simulink model "dribbel_v2"  (R2021b)
settings: Solver=FixedStepAuto  StartTime=0.0  StopTime=6  FixedStep=1e-4  MaxStep=1e-3  RelTol=1e-6
InitFcn:
  | dribbel_init_params;
values from neighbouring files (symbols this model uses):
  bd = [modifyPolynomial(polyder(b(1,:)),k); modifyPolynomial(polyder(b(2,:)),k)]    [trajectoryCostFun.m]
  D = m1*(Jvc1'*Jvc1)+m2*(Jvc2'*Jvc2)+m3*(Jvc3'*Jvc3)    [mass_matrix_planar_walker.m]
  g = 9.81    [create_robot_dribbel.m]
undefined symbols (not defined in the file or in its folder): bdd, c2, gamma, k, m, mH, q0, qd0, qdd0, xb
libraries: simulink x10
settings Model: Creator=moham  LastModifiedBy=moham
settings SolverCC: ShapePreserveControl=EnableAll  ZeroCrossAlgorithm=Adaptive

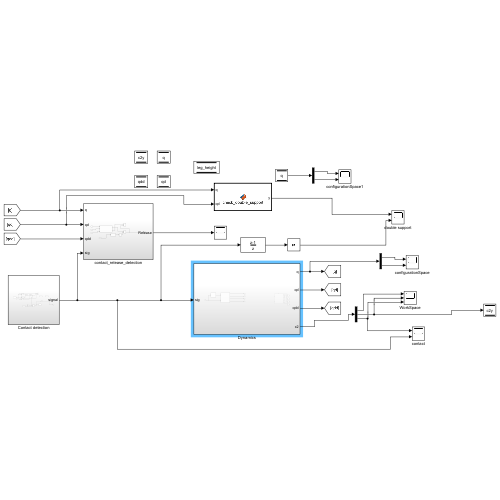
[thumbnail: Simulink's stored preview of the top-level diagram]
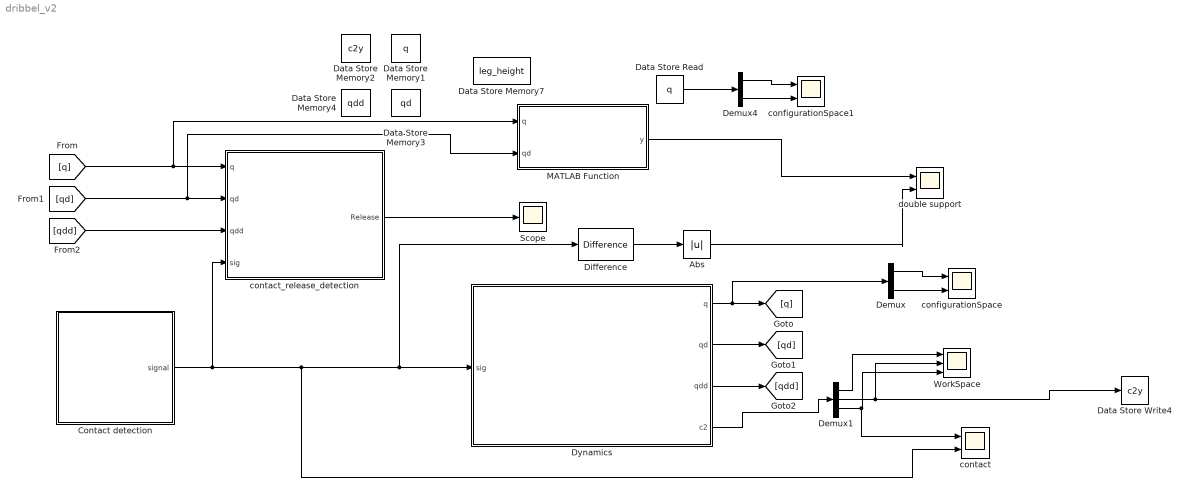
== system dribbel_v2 ==
  Abs : Abs
  Contact detection : Subsystem
  Data Store Memory1 : DataStoreMemory  DataStoreName=q  ReadBeforeWriteMsg=warning  WriteAfterWriteMsg=warning  WriteAfterReadMsg=warning  InitialValue=q0  ShowAdditionalParam=off
  Data Store Memory2 : DataStoreMemory  DataStoreName=c2y  ReadBeforeWriteMsg=warning  WriteAfterWriteMsg=warning  WriteAfterReadMsg=warning  InitialValue=c2(1,1)  ShowAdditionalParam=off
  Data Store Memory3 : DataStoreMemory  DataStoreName=qd  ReadBeforeWriteMsg=warning  WriteAfterWriteMsg=warning  WriteAfterReadMsg=warning  InitialValue=qd0  ShowAdditionalParam=off
  Data Store Memory4 : DataStoreMemory  DataStoreName=qdd  ReadBeforeWriteMsg=warning  WriteAfterWriteMsg=warning  WriteAfterReadMsg=warning  InitialValue=qd0  ShowAdditionalParam=off
  Data Store Memory7 : DataStoreMemory  DataStoreName=leg_height  ReadBeforeWriteMsg=warning  WriteAfterWriteMsg=warning  WriteAfterReadMsg=warning  ShowAdditionalParam=off
  Data Store Read : DataStoreRead  DataStoreName=q  IndexOptions=Index vector (dialog)  Indices=1  OutputSizes=1
  Data Store Write4 : DataStoreWrite  DataStoreName=c2y  IndexOptions=Index vector (dialog)  Indices=1  OutputSizes=1
  Demux : Demux  Outputs=2
  Demux1 : Demux  Outputs=3
  Demux4 : Demux  Outputs=2
  Difference : simulink/Discrete/Difference  ICPrevInput=0.0  OutMin=[]  OutMax=[]  OutDataType=fixdt(1, 16)  OutScaling=2^-10  DoSatur=off
  Dynamics : Subsystem
  MATLAB Function : MATLAB Function  TreatAsAtomicUnit=on
  Scope : Scope
  WorkSpace : Scope  NumInputPorts=3
  configurationSpace : Scope  NumInputPorts=2
  configurationSpace1 : Scope  NumInputPorts=2
  contact : Scope  NumInputPorts=2
  contact_release_detection : Subsystem
  double support : Scope  NumInputPorts=2
  wires:
  Demux1/1 -> WorkSpace/1
  Demux/2 -> configurationSpace/2
  Demux/1 -> configurationSpace/1
  Demux1/3 -> contact/1, WorkSpace/3
  Contact detection/1(signal) -> contact_release_detection/4(sig), contact/2, Difference/1, Dynamics/1(sig)
  Demux4/1 -> configurationSpace1/1
  Demux4/2 -> configurationSpace1/2
  Dynamics/1(q) -> Demux/1, [q]
  Dynamics/4(c2) -> Demux1/1
  Data Store Read/1 -> Demux4/1
  Demux1/2 -> WorkSpace/2, Data Store Write4/1
  Dynamics/2(qd) -> [qd]
  Dynamics/3(qdd) -> [qdd]
  [q] -> MATLAB Function/1(q), contact_release_detection/1(q)
  [qd] -> MATLAB Function/2(qd), contact_release_detection/2(qd)
  [qdd] -> contact_release_detection/3(qdd)
  contact_release_detection/1(Release) -> Scope/1
  MATLAB Function/1(y) -> double support/1
  Difference/1 -> Abs/1
  Abs/1 -> double support/2

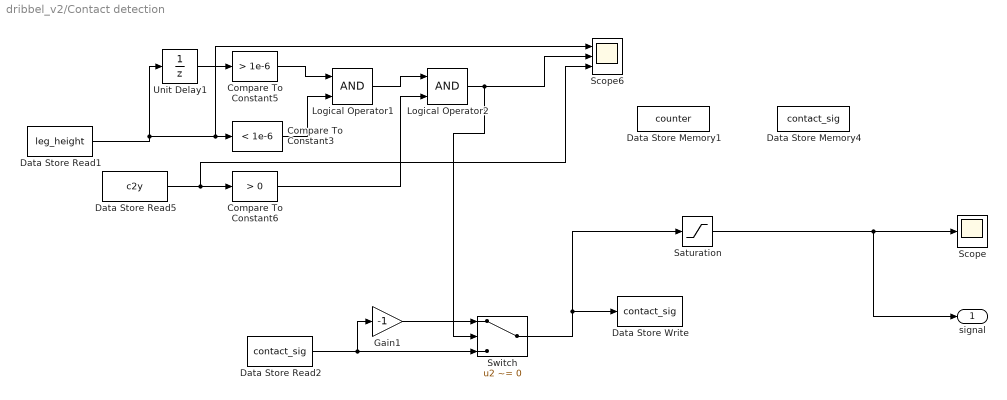
== system dribbel_v2/Contact detection ==
  Compare To Constant3 : simulink/Logic and Bit Operations/Compare To Constant  relop=<  const=1e-6  OutDataTypeStr=uint8  ZeroCross=off
  Compare To Constant5 : simulink/Logic and Bit Operations/Compare To Constant  relop=>  const=1e-6  OutDataTypeStr=uint8  ZeroCross=off
  Compare To Constant6 : simulink/Logic and Bit Operations/Compare To Constant  relop=>  const=0  OutDataTypeStr=uint8  ZeroCross=off
  Data Store Memory1 : DataStoreMemory  DataStoreName=counter  ReadBeforeWriteMsg=warning  WriteAfterWriteMsg=warning  WriteAfterReadMsg=warning  ShowAdditionalParam=off
  Data Store Memory4 : DataStoreMemory  DataStoreName=contact_sig  ReadBeforeWriteMsg=warning  WriteAfterWriteMsg=warning  WriteAfterReadMsg=warning  InitialValue=1  ShowAdditionalParam=off
  Data Store Read1 : DataStoreRead  DataStoreName=leg_height  IndexOptions=Index vector (dialog)  Indices=1  OutputSizes=1
  Data Store Read2 : DataStoreRead  DataStoreName=contact_sig  IndexOptions=Index vector (dialog)  Indices=1  OutputSizes=1
  Data Store Read5 : DataStoreRead  DataStoreName=c2y  IndexOptions=Index vector (dialog)  Indices=1  OutputSizes=1
  Data Store Write : DataStoreWrite  DataStoreName=contact_sig  IndexOptions=Index vector (dialog)  Indices=1  OutputSizes=1
  Gain1 : Gain  Gain=-1
  Logical Operator1 : Logic  AllPortsSameDT=off  OutDataTypeStr=boolean
  Logical Operator2 : Logic  AllPortsSameDT=off  OutDataTypeStr=boolean
  Saturation : Saturate  UpperLimit=1  LowerLimit=0  ZeroCross=off
  Scope : Scope
  Scope6 : Scope  NumInputPorts=3
  Switch : Switch  Criteria=u2 ~= 0  Threshold=0.5  ZeroCross=off
  Unit Delay1 : UnitDelay  SampleTime=-1  HasFrameUpgradeWarning=on
  signal : Outport
  wires:
  Gain1/1 -> Switch/1
  Data Store Read2/1 -> Gain1/1, Switch/3
  Switch/1 -> Saturation/1, Data Store Write/1
  Unit Delay1/1 -> Compare To Constant5/1
  Compare To Constant5/1 -> Logical Operator1/1
  Compare To Constant3/1 -> Logical Operator1/2
  Data Store Read5/1 -> Scope6/3, Compare To Constant6/1
  Compare To Constant6/1 -> Logical Operator2/2
  Logical Operator1/1 -> Logical Operator2/1
  Logical Operator2/1 -> Switch/2, Scope6/2
  Data Store Read1/1 -> Unit Delay1/1, Scope6/1, Compare To Constant3/1
  Saturation/1 -> signal/1, Scope/1

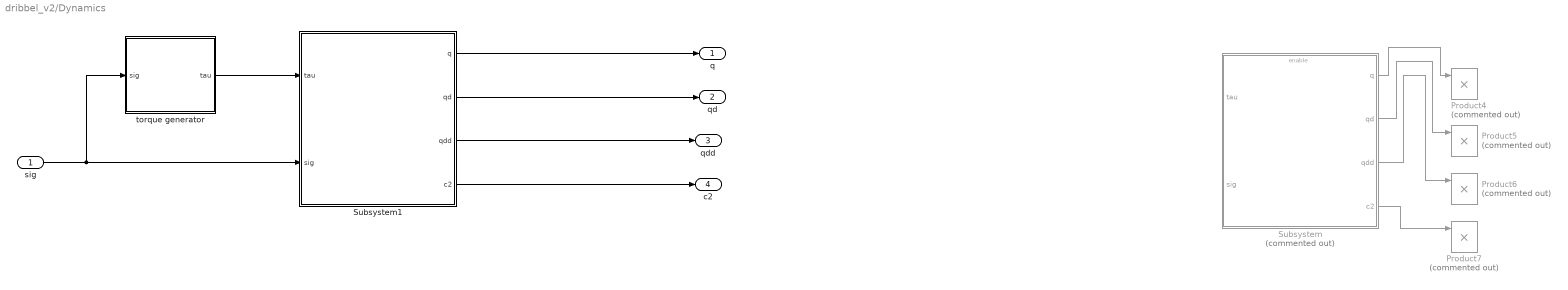
== system dribbel_v2/Dynamics ==
  sig : Inport
  Product{4..7} (4 alike) : Product  Commented=on
  Subsystem : Subsystem  Commented=on
  Subsystem1 : Subsystem
  torque generator : Subsystem
  q : Outport
  qd : Outport  Port=2
  qdd : Outport  Port=3
  c2 : Outport  Port=4
  wires:
  Subsystem1/1(q) -> q/1
  sig/1 -> torque generator/1(sig), Subsystem1/2(sig)
  Subsystem1/4(c2) -> c2/1
  Subsystem/1(q) -> Product4/1
  Subsystem/2(qd) -> Product5/1
  Subsystem/3(qdd) -> Product6/1
  Subsystem/4(c2) -> Product7/1
  Subsystem1/2(qd) -> qd/1
  Subsystem1/3(qdd) -> qdd/1
  torque generator/1(tau) -> Subsystem1/1(tau)

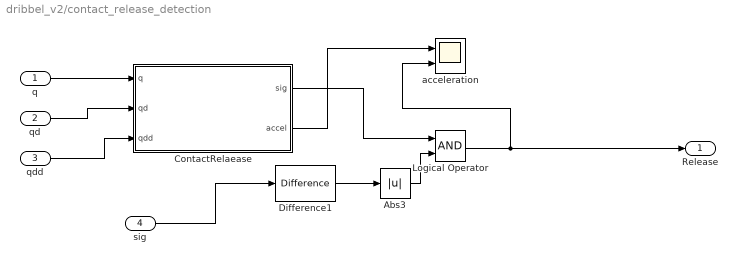
== system dribbel_v2/contact_release_detection ==
  q : Inport
  qd : Inport  Port=2
  qdd : Inport  Port=3
  sig : Inport  Port=4
  Abs3 : Abs
  ContactRelaease : Subsystem
  Difference1 : simulink/Discrete/Difference  ICPrevInput=0.0  OutMin=[]  OutMax=[]  OutDataType=fixdt(1, 16)  OutScaling=2^-10  DoSatur=off
  Logical Operator : Logic  AllPortsSameDT=off  OutDataTypeStr=boolean
  acceleration : Scope  NumInputPorts=2
  Release : Outport
  wires:
  Abs3/1 -> Logical Operator/2
  qd/1 -> ContactRelaease/2(qd)
  ContactRelaease/1(sig) -> Logical Operator/1
  q/1 -> ContactRelaease/1(q)
  Difference1/1 -> Abs3/1
  qdd/1 -> ContactRelaease/3(qdd)
  Logical Operator/1 -> acceleration/2, Release/1
  sig/1 -> Difference1/1
  ContactRelaease/2(accel) -> acceleration/1

== system dribbel_v2/Dynamics/Subsystem ==
  tau : Inport
  sig : Inport  Port=2
  Enable : EnablePort
  Dynamics1 : Subsystem
  Product : Product
  q : Outport
  qd : Outport  Port=2
  qdd : Outport  Port=3
  c2 : Outport  Port=4
  wires:
  Dynamics1/2(qd) -> qd/1
  Dynamics1/4(c2) -> c2/1
  tau/1 -> Dynamics1/2(tau)
  Dynamics1/3(qdd) -> qdd/1
  Dynamics1/1(q) -> Product/2
  Product/1 -> q/1
  sig/1 -> Product/1, Dynamics1/1(sig)

== system dribbel_v2/Dynamics/Subsystem1 ==
  tau : Inport
  sig : Inport  Port=2
  Dynamics : Subsystem
  q : Outport
  qd : Outport  Port=2
  qdd : Outport  Port=3
  c2 : Outport  Port=4
  wires:
  Dynamics/4(c2) -> c2/1
  tau/1 -> Dynamics/2(tau)
  Dynamics/2(qd) -> qd/1
  Dynamics/3(qdd) -> qdd/1
  Dynamics/1(q) -> q/1
  sig/1 -> Dynamics/1(sig)

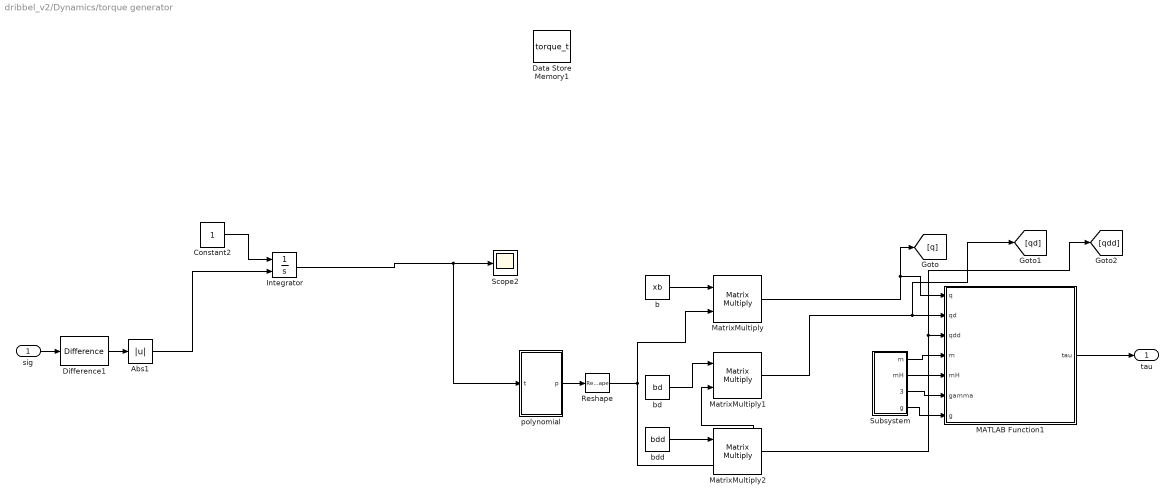
== system dribbel_v2/Dynamics/torque generator ==
  sig : Inport
  Abs1 : Abs
  Constant2 : Constant
  Data Store Memory1 : DataStoreMemory  DataStoreName=torque_t  ReadBeforeWriteMsg=warning  WriteAfterWriteMsg=warning  WriteAfterReadMsg=warning  ShowAdditionalParam=off
  Difference1 : simulink/Discrete/Difference  ICPrevInput=1  OutMin=[]  OutMax=[]  OutDataType=fixdt(1, 16)  OutScaling=2^-10  DoSatur=off
  Integrator : Integrator  ExternalReset=rising
  MATLAB Function1 : MATLAB Function  TreatAsAtomicUnit=on
  MatrixMultiply : Product  Multiplication=Matrix(*)
  MatrixMultiply1 : Product  Multiplication=Matrix(*)
  MatrixMultiply2 : Product  Multiplication=Matrix(*)
  Reshape : Reshape  OutputDimensionality=Column vector (2-D)
  Scope2 : Scope
  Subsystem : Subsystem
  b : Constant  Value=xb
  bd : Constant  Value=bd
  bdd : Constant  Value=bdd
  polynomial : Subsystem
  tau : Outport
  wires:
  bd/1 -> MatrixMultiply1/1
  bdd/1 -> MatrixMultiply2/1
  b/1 -> MatrixMultiply/1
  Subsystem/1(m) -> MATLAB Function1/4(m)
  Subsystem/2(mH) -> MATLAB Function1/5(mH)
  Subsystem/3(gamma) -> MATLAB Function1/6(gamma)
  Subsystem/4(g) -> MATLAB Function1/7(g)
  Reshape/1 -> MatrixMultiply/2, MatrixMultiply1/2, MatrixMultiply2/2
  polynomial/1(p) -> Reshape/1
  sig/1 -> Difference1/1
  Difference1/1 -> Abs1/1
  Abs1/1 -> Integrator/2
  MATLAB Function1/1(tau) -> tau/1
  MatrixMultiply/1 -> [q], MATLAB Function1/1(q)
  MatrixMultiply1/1 -> [qd], MATLAB Function1/2(qd)
  MatrixMultiply2/1 -> [qdd], MATLAB Function1/3(qdd)
  Integrator/1 -> polynomial/1(t), Scope2/1
  Constant2/1 -> Integrator/1

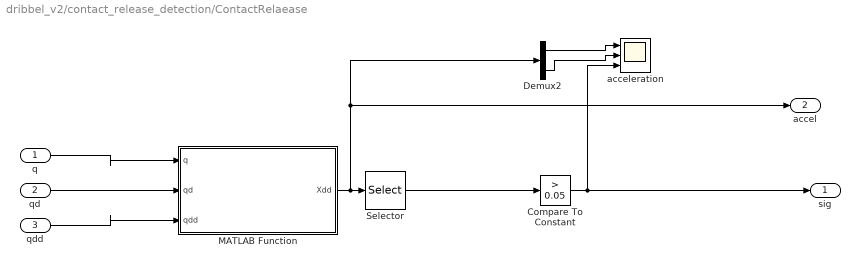
== system dribbel_v2/contact_release_detection/ContactRelaease ==
  q : Inport
  qd : Inport  Port=2
  qdd : Inport  Port=3
  Compare To Constant : simulink/Logic and Bit Operations/Compare To Constant  relop=>  const=0.05  OutDataTypeStr=boolean
  Demux2 : Demux  Outputs=2
  MATLAB Function : MATLAB Function  TreatAsAtomicUnit=on
  Selector : Selector  InputPortWidth=2  IndexOptions=Index vector (dialog)  Indices=2  OutputSizes=1
  acceleration : Scope  NumInputPorts=3
  sig : Outport
  accel : Outport  Port=2
  wires:
  qd/1 -> MATLAB Function/2(qd)
  qdd/1 -> MATLAB Function/3(qdd)
  q/1 -> MATLAB Function/1(q)
  MATLAB Function/1(Xdd) -> accel/1, Demux2/1, Selector/1
  Selector/1 -> Compare To Constant/1
  Demux2/1 -> acceleration/1
  Demux2/2 -> acceleration/2
  Compare To Constant/1 -> sig/1, acceleration/3

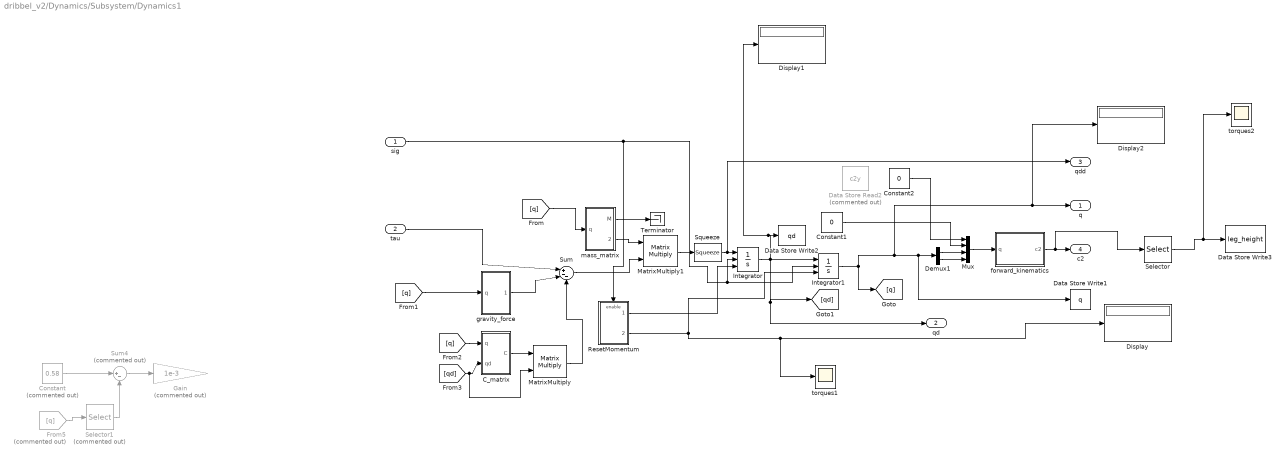
== system dribbel_v2/Dynamics/Subsystem/Dynamics1 ==
  sig : Inport
  tau : Inport  Port=2
  C_matrix : Subsystem
  Constant : Constant  Commented=on  Value=0.58
  Constant1 : Constant  Value=0
  Constant2 : Constant  Value=0
  Data Store Read2 : DataStoreRead  Commented=on  DataStoreName=c2y  IndexOptions=Index vector (dialog)  Indices=1  OutputSizes=1
  Data Store Write1 : DataStoreWrite  DataStoreName=q  IndexOptions=Index vector (dialog)  Indices=1  OutputSizes=1
  Data Store Write2 : DataStoreWrite  DataStoreName=qd  IndexOptions=Index vector (dialog)  Indices=1  OutputSizes=1
  Data Store Write3 : DataStoreWrite  DataStoreName=leg_height  IndexOptions=Index vector (dialog)  Indices=1  OutputSizes=1
  Demux1 : Demux  Outputs=2
  Display : Display
  Display1 : Display
  Display2 : Display
  From5 : From  Commented=on  GotoTag=q
  Gain : Gain  Commented=on  Gain=1e-3
  Integrator : Integrator  ExternalReset=rising  InitialConditionSource=external  InitialCondition=qd0
  Integrator1 : Integrator  ExternalReset=rising  InitialConditionSource=external  InitialCondition=q0
  MatrixMultiply : Product  Multiplication=Matrix(*)
  MatrixMultiply1 : Product  Multiplication=Matrix(*)
  Mux : Mux
  ResetMomentum : Subsystem
  Selector : Selector  InputPortWidth=3  IndexOptions=Index vector (dialog)  Indices=3  OutputSizes=1
  Selector1 : Selector  Commented=on  InputPortWidth=2  IndexOptions=Index vector (dialog)  Indices=2  OutputSizes=1
  Squeeze : Squeeze
  Sum : Sum  Inputs=|+--
  Sum4 : Sum  Commented=on  Inputs=|+-
  Terminator : Terminator
  forward_kinematics : MATLAB Function  TreatAsAtomicUnit=on
  gravity_force : Subsystem
  mass_matrix : Subsystem
  torques1 : Scope
  torques2 : Scope
  q : Outport
  qd : Outport  Port=2
  qdd : Outport  Port=3
  c2 : Outport  Port=4
  wires:
  Constant2/1 -> Mux/1
  C_matrix/1(C) -> MatrixMultiply/1
  mass_matrix/1(M) -> Terminator/1
  mass_matrix/2(M_inv) -> MatrixMultiply1/1
  Sum/1 -> MatrixMultiply1/2
  gravity_force/1(dvdq) -> Sum/2
  MatrixMultiply1/1 -> Squeeze/1
  [qd] -> MatrixMultiply/2, C_matrix/2(qd)
  [q] -> mass_matrix/1(q)
  [q] -> C_matrix/1(q)
  MatrixMultiply/1 -> Sum/3
  [q] -> gravity_force/1(q)
  Squeeze/1 -> Integrator/1, qdd/1
  Demux1/2 -> Mux/4
  Demux1/1 -> Mux/3
  forward_kinematics/1(c2) -> Selector/1, c2/1
  Integrator/1 -> qd/1, [qd], Display1/1, Data Store Write2/1, Integrator1/1
  Mux/1 -> forward_kinematics/1(q)
  Integrator1/1 -> [q], Display2/1, q/1, Demux1/1, Data Store Write1/1
  Selector/1 -> torques2/1, Data Store Write3/1
  Constant1/1 -> Mux/2
  Selector1/1 -> Sum4/2
  From5/1 -> Selector1/1
  Sum4/1 -> Gain/1
  Constant/1 -> Sum4/1
  tau/1 -> Sum/1
  ResetMomentum/2(q_new) -> Integrator1/3, Display/1, torques1/1
  sig/1 -> ResetMomentum/Enable, Integrator1/2, Integrator/2
  ResetMomentum/1(qd_new) -> Integrator/3

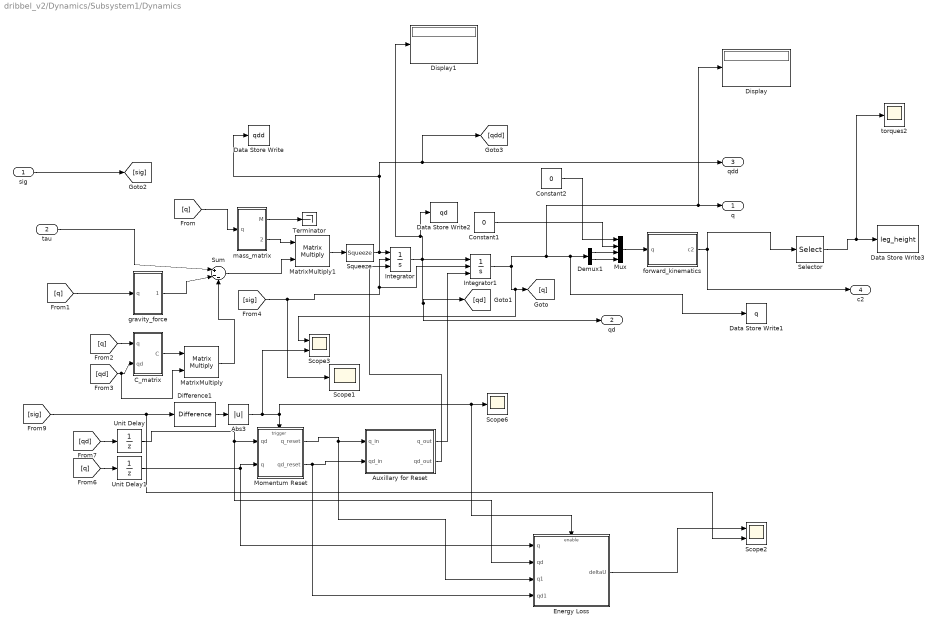
== system dribbel_v2/Dynamics/Subsystem1/Dynamics ==
  sig : Inport
  tau : Inport  Port=2
  Abs3 : Abs
  Auxillary for Reset : Subsystem
  C_matrix : Subsystem
  Constant1 : Constant  Value=0
  Constant2 : Constant  Value=0
  Data Store Write : DataStoreWrite  DataStoreName=qdd  IndexOptions=Index vector (dialog)  Indices=1  OutputSizes=1
  Data Store Write1 : DataStoreWrite  DataStoreName=q  IndexOptions=Index vector (dialog)  Indices=1  OutputSizes=1
  Data Store Write2 : DataStoreWrite  DataStoreName=qd  IndexOptions=Index vector (dialog)  Indices=1  OutputSizes=1
  Data Store Write3 : DataStoreWrite  DataStoreName=leg_height  IndexOptions=Index vector (dialog)  Indices=1  OutputSizes=1
  Demux1 : Demux  Outputs=2
  Difference1 : simulink/Discrete/Difference  ICPrevInput=0.0  OutMin=[]  OutMax=[]  OutDataType=fixdt(1, 16)  OutScaling=2^-10  DoSatur=off
  Display : Display
  Display1 : Display
  Energy Loss : Subsystem  TreatAsAtomicUnit=on
  Integrator : Integrator  ExternalReset=either  InitialConditionSource=external  InitialCondition=qd0  ZeroCross=off
  Integrator1 : Integrator  ExternalReset=either  InitialConditionSource=external  InitialCondition=q0
  MatrixMultiply : Product  Multiplication=Matrix(*)
  MatrixMultiply1 : Product  Multiplication=Matrix(*)
  Momentum Reset : Subsystem
  Mux : Mux
  Scope1 : Scope
  Scope2 : Scope  NumInputPorts=2
  Scope3 : Scope  NumInputPorts=2
  Scope6 : Scope
  Selector : Selector  InputPortWidth=3  IndexOptions=Index vector (dialog)  Indices=3  OutputSizes=1
  Squeeze : Squeeze
  Sum : Sum  Inputs=|+--
  Terminator : Terminator
  Unit Delay : UnitDelay  InitialCondition=qd0  SampleTime=-1  HasFrameUpgradeWarning=on
  Unit Delay1 : UnitDelay  InitialCondition=q0  SampleTime=-1  HasFrameUpgradeWarning=on
  forward_kinematics : MATLAB Function  TreatAsAtomicUnit=on
  gravity_force : Subsystem
  mass_matrix : Subsystem
  torques2 : Scope
  q : Outport
  qd : Outport  Port=2
  qdd : Outport  Port=3
  c2 : Outport  Port=4
  wires:
  tau/1 -> Sum/1
  Constant1/1 -> Mux/2
  Selector/1 -> Data Store Write3/1, torques2/1
  Mux/1 -> forward_kinematics/1(q)
  Integrator/1 -> Integrator1/1, Data Store Write2/1, Display1/1, [qd], qd/1
  forward_kinematics/1(c2) -> c2/1, Selector/1
  Demux1/1 -> Mux/3
  Demux1/2 -> Mux/4
  Squeeze/1 -> Data Store Write/1, [qdd], qdd/1, Integrator/1
  [q] -> gravity_force/1(q)
  MatrixMultiply/1 -> Sum/3
  [q] -> C_matrix/1(q)
  [q] -> mass_matrix/1(q)
  [qd] -> C_matrix/2(qd), MatrixMultiply/2
  MatrixMultiply1/1 -> Squeeze/1
  gravity_force/1(dvdq) -> Sum/2
  Sum/1 -> MatrixMultiply1/2
  mass_matrix/2(M_inv) -> MatrixMultiply1/1
  mass_matrix/1(M) -> Terminator/1
  C_matrix/1(C) -> MatrixMultiply/1
  Constant2/1 -> Mux/1
  Integrator1/1 -> Data Store Write1/1, Demux1/1, q/1, Display/1, Scope3/1, [q]
  sig/1 -> [sig]
  [q] -> Unit Delay1/1
  [sig] -> Scope2/2, Difference1/1
  Difference1/1 -> Abs3/1
  Momentum Reset/1(q_reset) -> Energy Loss/3(q1), Auxillary for Reset/1(q_in)
  Auxillary for Reset/1(q_out) -> Integrator1/3
  Auxillary for Reset/2(qd_out) -> Integrator/3
  [sig] -> Scope1/1, Integrator1/2, Integrator/2
  Unit Delay/1 -> Energy Loss/2(qd), Momentum Reset/1(qd)
  Unit Delay1/1 -> Momentum Reset/2(q), Energy Loss/1(q)
  [qd] -> Unit Delay/1
  Energy Loss/1(deltaU) -> Scope2/1
  Momentum Reset/2(qd_reset) -> Auxillary for Reset/2(qd_in), Energy Loss/4(qd1)
  Abs3/1 -> Scope3/2, Energy Loss/Enable, Scope6/1, Momentum Reset/Trigger

== system dribbel_v2/Dynamics/torque generator/Subsystem ==
  Constan2 : Constant  Value=mH
  Constant : Constant  Value=g
  Constant1 : Constant  Value=gamma
  leg_mass2 : Constant  Value=m
  m : Outport
  mH : Outport  Port=2
  gamma : Outport  Port=3
  g : Outport  Port=4
  wires:
  Constan2/1 -> mH/1
  Constant1/1 -> gamma/1
  Constant/1 -> g/1
  leg_mass2/1 -> m/1

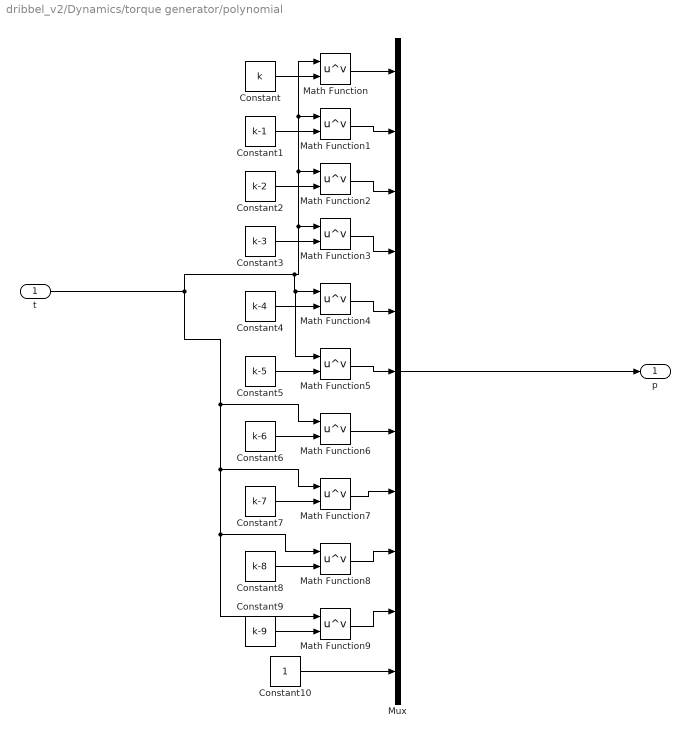
== system dribbel_v2/Dynamics/torque generator/polynomial ==
  t : Inport
  Constant : Constant  Value=k
  Constant1 : Constant  Value=k-1
  Constant10 : Constant
  Constant2 : Constant  Value=k-2
  Constant3 : Constant  Value=k-3
  Constant4 : Constant  Value=k-4
  Constant5 : Constant  Value=k-5
  Constant6 : Constant  Value=k-6
  Constant7 : Constant  Value=k-7
  Constant8 : Constant  Value=k-8
  Constant9 : Constant  Value=k-9
  Math Function{,1..9} (10 alike) : Math  Operator=pow  SaturateOnIntegerOverflow=on
  Mux : Mux  Inputs=11
  p : Outport
  wires:
  Constant/1 -> Math Function/2
  Constant1/1 -> Math Function1/2
  Constant2/1 -> Math Function2/2
  Constant3/1 -> Math Function3/2
  Constant4/1 -> Math Function4/2
  Constant5/1 -> Math Function5/2
  Constant6/1 -> Math Function6/2
  Constant7/1 -> Math Function7/2
  Constant8/1 -> Math Function8/2
  Constant9/1 -> Math Function9/2
  t/1 -> Math Function5/1, Math Function4/1, Math Function3/1, Math Function2/1, Math Function1/1, Math Function/1, Math Function9/1, Math Function8/1, Math Function7/1, Math Function6/1
  Math Function/1 -> Mux/1
  Math Function1/1 -> Mux/2
  Math Function2/1 -> Mux/3
  Math Function3/1 -> Mux/4
  Math Function4/1 -> Mux/5
  Math Function5/1 -> Mux/6
  Math Function6/1 -> Mux/7
  Math Function7/1 -> Mux/8
  Math Function8/1 -> Mux/9
  Math Function9/1 -> Mux/10
  Mux/1 -> p/1
  Constant10/1 -> Mux/11

== system dribbel_v2/Dynamics/Subsystem/Dynamics1/C_matrix ==
  q : Inport
  qd : Inport  Port=2
  C_matrix : MATLAB Function  TreatAsAtomicUnit=on
  leg_mass1 : Constant  Value=m
  C : Outport
  wires:
  leg_mass1/1 -> C_matrix/3(m)
  C_matrix/1(C) -> C/1
  q/1 -> C_matrix/1(q)
  qd/1 -> C_matrix/2(qd)

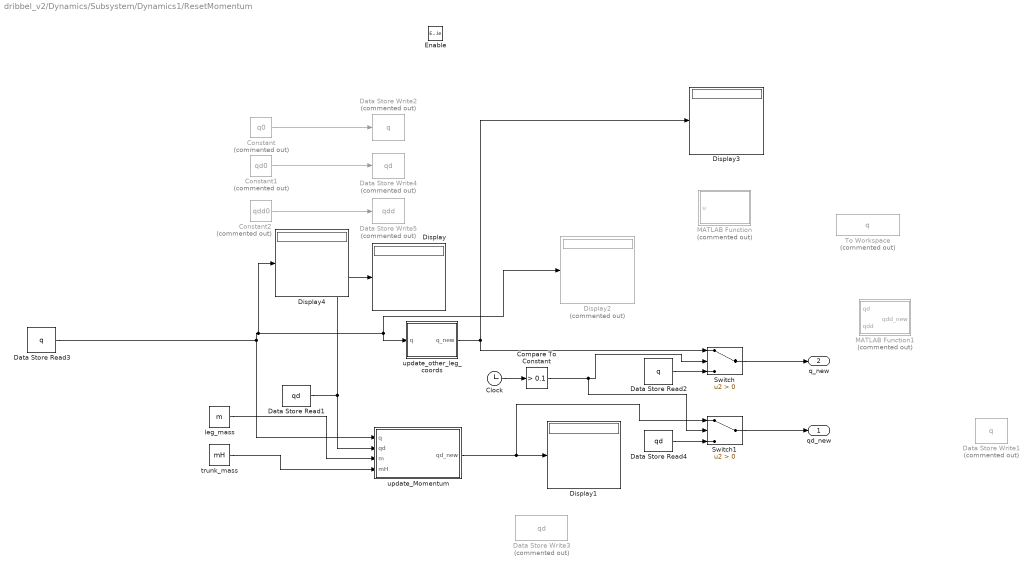
== system dribbel_v2/Dynamics/Subsystem/Dynamics1/ResetMomentum ==
  Enable : EnablePort  StatesWhenEnabling=reset  ZeroCross=off
  Clock : Clock
  Compare To Constant : simulink/Logic and Bit Operations/Compare To Constant  relop=>  const=0.1  OutDataTypeStr=boolean
  Constant : Constant  Commented=on  Value=q0
  Constant1 : Constant  Commented=on  Value=qd0
  Constant2 : Constant  Commented=on  Value=qdd0
  Data Store Read1 : DataStoreRead  DataStoreName=qd  IndexOptions=Index vector (dialog)  Indices=1  OutputSizes=1
  Data Store Read2 : DataStoreRead  DataStoreName=q  IndexOptions=Index vector (dialog)  Indices=1  OutputSizes=1
  Data Store Read3 : DataStoreRead  DataStoreName=q  IndexOptions=Index vector (dialog)  Indices=1  OutputSizes=1
  Data Store Read4 : DataStoreRead  DataStoreName=qd  IndexOptions=Index vector (dialog)  Indices=1  OutputSizes=1
  Data Store Write1 : DataStoreWrite  Commented=on  DataStoreName=q  IndexOptions=Index vector (dialog)  Indices=1  OutputSizes=1
  Data Store Write2 : DataStoreWrite  Commented=on  DataStoreName=q  IndexOptions=Index vector (dialog)  Indices=1  OutputSizes=1
  Data Store Write3 : DataStoreWrite  Commented=on  DataStoreName=qd  IndexOptions=Index vector (dialog)  Indices=1  OutputSizes=1
  Data Store Write4 : DataStoreWrite  Commented=on  DataStoreName=qd  IndexOptions=Index vector (dialog)  Indices=1  OutputSizes=1
  Data Store Write5 : DataStoreWrite  Commented=on  DataStoreName=qdd  IndexOptions=Index vector (dialog)  Indices=1  OutputSizes=1
  Display{,1,3..4} (4 alike) : Display
  Display2 : Display  Commented=on
  MATLAB Function : MATLAB Function  Commented=on  TreatAsAtomicUnit=on
  MATLAB Function1 : MATLAB Function  Commented=on  TreatAsAtomicUnit=on
  Switch : Switch  Criteria=u2 > Threshold
  Switch1 : Switch  Criteria=u2 > Threshold
  To Workspace : ToWorkspace  Commented=on  VariableName=q  SaveFormat=Timeseries  SampleTime=-1
  leg_mass : Constant  Value=m
  trunk_mass : Constant  Value=mH
  update_Momentum : MATLAB Function  TreatAsAtomicUnit=on
  update_other_leg_coords : MATLAB Function  TreatAsAtomicUnit=on
  qd_new : Outport
  q_new : Outport  Port=2
  wires:
  update_Momentum/1(qd_new) -> Switch1/1, Display1/1
  update_other_leg_coords/1(q_new) -> Display3/1, Switch/1
  Constant2/1 -> Data Store Write5/1
  Constant1/1 -> Data Store Write4/1
  Constant/1 -> Data Store Write2/1
  leg_mass/1 -> update_Momentum/3(m)
  Data Store Read1/1 -> update_Momentum/2(qd), Display/1
  trunk_mass/1 -> update_Momentum/4(mH)
  Data Store Read2/1 -> Switch/3
  Switch1/1 -> qd_new/1
  Data Store Read4/1 -> Switch1/3
  Clock/1 -> Compare To Constant/1
  Compare To Constant/1 -> Switch1/2, Switch/2
  Switch/1 -> q_new/1
  Data Store Read3/1 -> Display4/1, update_other_leg_coords/1(q), Display2/1, update_Momentum/1(q)

== system dribbel_v2/Dynamics/Subsystem/Dynamics1/gravity_force ==
  q : Inport
  Constant : Constant  Value=g
  Graitational_Force : MATLAB Function  TreatAsAtomicUnit=on
  gamma : Constant  Value=gamma
  leg_mass2 : Constant  Value=m
  trunk_mass2 : Constant  Value=mH
  dvdq : Outport
  wires:
  trunk_mass2/1 -> Graitational_Force/3(mH)
  leg_mass2/1 -> Graitational_Force/2(m)
  gamma/1 -> Graitational_Force/4(gamma)
  Graitational_Force/1(dvdq) -> dvdq/1
  q/1 -> Graitational_Force/1(q)
  Constant/1 -> Graitational_Force/5(g)

== system dribbel_v2/Dynamics/Subsystem/Dynamics1/mass_matrix ==
  q : Inport
  Mass_Matrix : MATLAB Function  TreatAsAtomicUnit=on
  leg_mass : Constant  Value=m
  trunk_mass : Constant  Value=mH
  M : Outport
  M_inv : Outport  Port=2
  wires:
  Mass_Matrix/2(M_inv) -> M_inv/1
  leg_mass/1 -> Mass_Matrix/2(m)
  q/1 -> Mass_Matrix/1(q)
  Mass_Matrix/1(M) -> M/1
  trunk_mass/1 -> Mass_Matrix/3(mH)

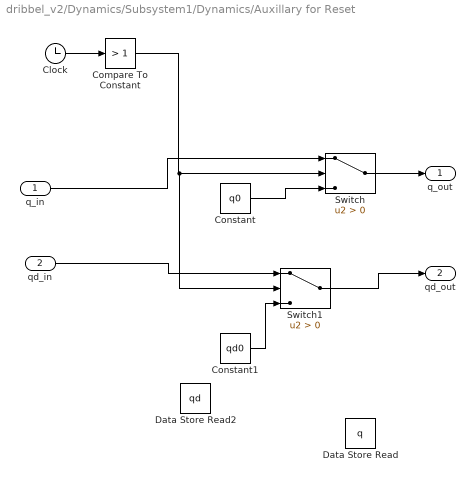
== system dribbel_v2/Dynamics/Subsystem1/Dynamics/Auxillary for Reset ==
  q_in : Inport
  qd_in : Inport  Port=2
  Clock : Clock
  Compare To Constant : simulink/Logic and Bit Operations/Compare To Constant  relop=>  const=1  OutDataTypeStr=boolean
  Constant : Constant  Value=q0
  Constant1 : Constant  Value=qd0
  Data Store Read : DataStoreRead  DataStoreName=q  IndexOptions=Index vector (dialog)  Indices=1  OutputSizes=1
  Data Store Read2 : DataStoreRead  DataStoreName=qd  IndexOptions=Index vector (dialog)  Indices=1  OutputSizes=1
  Switch : Switch  Criteria=u2 > Threshold
  Switch1 : Switch  Criteria=u2 > Threshold
  q_out : Outport
  qd_out : Outport  Port=2
  wires:
  Clock/1 -> Compare To Constant/1
  q_in/1 -> Switch/1
  Compare To Constant/1 -> Switch1/2, Switch/2
  qd_in/1 -> Switch1/1
  Constant/1 -> Switch/3
  Constant1/1 -> Switch1/3
  Switch/1 -> q_out/1
  Switch1/1 -> qd_out/1

== system dribbel_v2/Dynamics/Subsystem1/Dynamics/C_matrix ==
  q : Inport
  qd : Inport  Port=2
  C_matrix : MATLAB Function  TreatAsAtomicUnit=on
  leg_mass1 : Constant  Value=m
  C : Outport
  wires:
  qd/1 -> C_matrix/2(qd)
  q/1 -> C_matrix/1(q)
  C_matrix/1(C) -> C/1
  leg_mass1/1 -> C_matrix/3(m)

== system dribbel_v2/Dynamics/Subsystem1/Dynamics/Energy Loss ==
  q : Inport
  qd : Inport  Port=2
  q1 : Inport  Port=3
  qd1 : Inport  Port=4
  Enable : EnablePort
  Energy After impact : MATLAB Function  TreatAsAtomicUnit=on
  Energy before impact : MATLAB Function  TreatAsAtomicUnit=on
  Sum : Sum  Inputs=-+|
  deltaU : Outport
  wires:
  q/1 -> Energy before impact/1(q)
  qd/1 -> Energy before impact/2(qd)
  Energy before impact/1(K) -> Sum/1
  qd1/1 -> Energy After impact/2(qd)
  q1/1 -> Energy After impact/1(q)
  Energy After impact/1(K) -> Sum/2
  Sum/1 -> deltaU/1

== system dribbel_v2/Dynamics/Subsystem1/Dynamics/Momentum Reset ==
  qd : Inport
  q : Inport  Port=2
  Trigger : TriggerPort  VariantControl=(inherit)  ZeroCross=off  PortDimensions=1
  Display2 : Display
  Display3 : Display
  ResetMomentum : Subsystem
  q_reset : Outport
  qd_reset : Outport  Port=2
  wires:
  ResetMomentum/1(qd_new) -> qd_reset/1, Display3/1
  ResetMomentum/2(q_new) -> q_reset/1, Display2/1
  qd/1 -> ResetMomentum/1(qd)
  q/1 -> ResetMomentum/2(q)

== system dribbel_v2/Dynamics/Subsystem1/Dynamics/gravity_force ==
  q : Inport
  Constant : Constant  Value=g
  Graitational_Force : MATLAB Function  TreatAsAtomicUnit=on
  gamma : Constant  Value=gamma
  leg_mass2 : Constant  Value=m
  trunk_mass2 : Constant  Value=mH
  dvdq : Outport
  wires:
  Constant/1 -> Graitational_Force/5(g)
  q/1 -> Graitational_Force/1(q)
  Graitational_Force/1(dvdq) -> dvdq/1
  gamma/1 -> Graitational_Force/4(gamma)
  leg_mass2/1 -> Graitational_Force/2(m)
  trunk_mass2/1 -> Graitational_Force/3(mH)

== system dribbel_v2/Dynamics/Subsystem1/Dynamics/mass_matrix ==
  q : Inport
  Mass_Matrix : MATLAB Function  TreatAsAtomicUnit=on
  leg_mass : Constant  Value=m
  trunk_mass : Constant  Value=mH
  M : Outport
  M_inv : Outport  Port=2
  wires:
  trunk_mass/1 -> Mass_Matrix/3(mH)
  Mass_Matrix/1(M) -> M/1
  q/1 -> Mass_Matrix/1(q)
  leg_mass/1 -> Mass_Matrix/2(m)
  Mass_Matrix/2(M_inv) -> M_inv/1

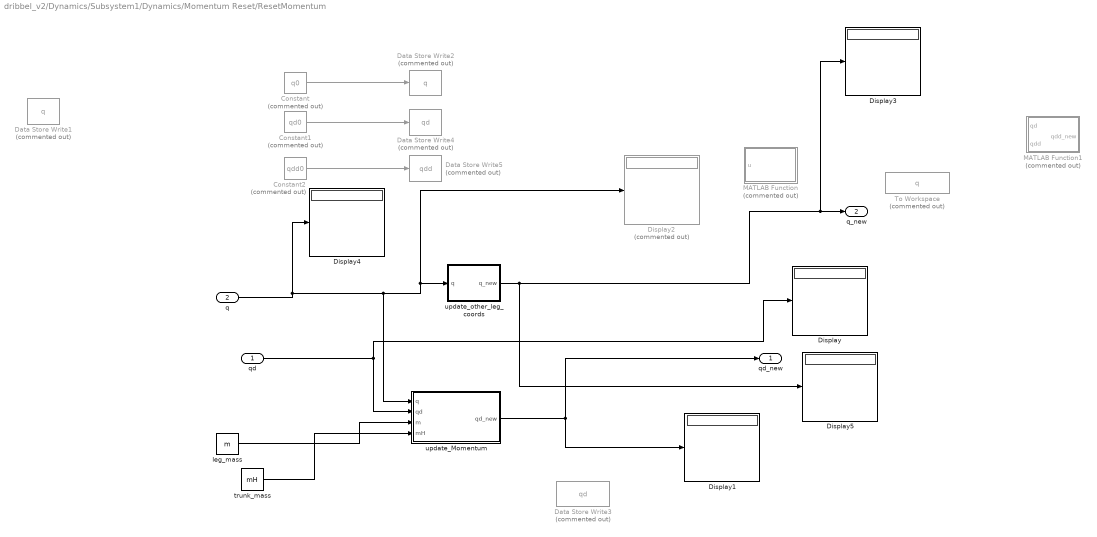
== system dribbel_v2/Dynamics/Subsystem1/Dynamics/Momentum Reset/ResetMomentum ==
  qd : Inport
  q : Inport  Port=2
  Constant : Constant  Commented=on  Value=q0
  Constant1 : Constant  Commented=on  Value=qd0
  Constant2 : Constant  Commented=on  Value=qdd0
  Data Store Write1 : DataStoreWrite  Commented=on  DataStoreName=q  IndexOptions=Index vector (dialog)  Indices=1  OutputSizes=1
  Data Store Write2 : DataStoreWrite  Commented=on  DataStoreName=q  IndexOptions=Index vector (dialog)  Indices=1  OutputSizes=1
  Data Store Write3 : DataStoreWrite  Commented=on  DataStoreName=qd  IndexOptions=Index vector (dialog)  Indices=1  OutputSizes=1
  Data Store Write4 : DataStoreWrite  Commented=on  DataStoreName=qd  IndexOptions=Index vector (dialog)  Indices=1  OutputSizes=1
  Data Store Write5 : DataStoreWrite  Commented=on  DataStoreName=qdd  IndexOptions=Index vector (dialog)  Indices=1  OutputSizes=1
  Display{,1,3..5} (5 alike) : Display
  Display2 : Display  Commented=on
  MATLAB Function : MATLAB Function  Commented=on  TreatAsAtomicUnit=on
  MATLAB Function1 : MATLAB Function  Commented=on  TreatAsAtomicUnit=on
  To Workspace : ToWorkspace  Commented=on  VariableName=q  SaveFormat=Timeseries  SampleTime=-1
  leg_mass : Constant  Value=m
  trunk_mass : Constant  Value=mH
  update_Momentum : MATLAB Function  TreatAsAtomicUnit=on
  update_other_leg_coords : MATLAB Function  TreatAsAtomicUnit=on
  qd_new : Outport
  q_new : Outport  Port=2
  wires:
  Constant2/1 -> Data Store Write5/1
  Constant1/1 -> Data Store Write4/1
  Constant/1 -> Data Store Write2/1
  leg_mass/1 -> update_Momentum/3(m)
  q/1 -> Display4/1, update_Momentum/1(q), update_other_leg_coords/1(q), Display2/1
  trunk_mass/1 -> update_Momentum/4(mH)
  update_Momentum/1(qd_new) -> qd_new/1, Display1/1
  update_other_leg_coords/1(q_new) -> Display3/1, q_new/1, Display5/1
  qd/1 -> update_Momentum/2(qd), Display/1

== matlab function dribbel_v2/Dynamics/Subsystem1/Dynamics/Momentum Reset/ResetMomentum/MATLAB Function ==
  data: u input
function fcn(u)

if u > 0
    run('dribbel_init_params');
end

== matlab function dribbel_v2/Dynamics/Subsystem1/Dynamics/Momentum Reset/ResetMomentum/MATLAB Function1 ==
  data: qd input; qdd_new output; qdd input
function qdd_new = chagne_Sign(qd,qdd)

qdd_new(1) = sign(qd(1))*

y = u;

== matlab function dribbel_v2/Dynamics/Subsystem1/Dynamics/Momentum Reset/ResetMomentum/update_Momentum ==
  data: q input; qd_new output; qd input; m input; mH input
function qd_new = MomentumReset(q,qd,m,mH)

MPM = [(-m-2*m*cos(2*q(1))+4*(m+mH)*cos(4*q(1)))/(3*m+4*mH-2*m*cos(4*q(1))),                 (-2*m*cos(2*q(1)))/(3*m+4*mH-2*m*cos(4*q(1)));
       (8*(m+mH)*(1+2*cos(2*q(1)))*sin(q(1))^2)/(3*m+4*mH-2*m*cos(4*q(1))),                  (-m+2*m*cos(2*q(1)))/(3*m+4*mH-2*m*cos(4*q(1)))];
% [~,jacc] = relabelled_coords(q);

qd_new = MPM*qd;

== matlab function dribbel_v2/Dynamics/Subsystem1/Dynamics/C_matrix/C_matrix ==
  data: q input size=[2,1]; C output size=[2,2]; qd input size=[2,1]; m input
function C = create_C(q, qd,m)

c11 = 0.0;
c12 = ((3/4)*qd(1)+qd(2)/2)*m*sin(q(2));
c21 = -(qd(1)/2 + qd(2)/4)*m*sin(q(2));
c22 = 0.0;
C = [c11 c12; c21 c22];

end

== matlab function dribbel_v2/Dynamics/Subsystem1/Dynamics/Momentum Reset/ResetMomentum/update_other_leg_coords ==
  data: q input; q_new output
function q_new = fcn(q)

% q1 = q(1)-sin(q(3))+sin(q(3)+q(4));
% q2 = q(2)+cos(q(3))-cos(q(3)+q(4));
q3 = q(1)+q(2);
q4 = -q(2);
q_new = [q3 q4]';

== matlab function dribbel_v2/Dynamics/Subsystem/Dynamics1/ResetMomentum/MATLAB Function ==
  data: u input
function fcn(u)

if u > 0
    run('dribbel_init_params');
end

== matlab function dribbel_v2/Dynamics/Subsystem/Dynamics1/ResetMomentum/MATLAB Function1 ==
  data: qd input; qdd_new output; qdd input
function qdd_new = chagne_Sign(qd,qdd)

qdd_new(1) = sign(qd(1))*

y = u;

== matlab function dribbel_v2/Dynamics/Subsystem/Dynamics1/ResetMomentum/update_Momentum ==
  data: q input; qd_new output; qd input; m input; mH input
function qd_new = MomentumReset(q,qd,m,mH)

MPM = [(-m-2*m*cos(2*q(1))+4*(m+mH)*cos(4*q(1)))/(3*m+4*mH-2*m*cos(4*q(1))),                 (-2*m*cos(2*q(1)))/(3*m+4*mH-2*m*cos(4*q(1)));
       (8*(m+mH)*(1+2*cos(2*q(1)))*sin(q(1))^2)/(3*m+4*mH-2*m*cos(4*q(1))),                  (-m+2*m*cos(2*q(1)))/(3*m+4*mH-2*m*cos(4*q(1)))];
% [~,jacc] = relabelled_coords(q);

qd_new = MPM*qd;

== matlab function dribbel_v2/Dynamics/Subsystem/Dynamics1/ResetMomentum/update_other_leg_coords ==
  data: q input; q_new output
function q_new = fcn(q)

% q1 = q(1)-sin(q(3))+sin(q(3)+q(4));
% q2 = q(2)+cos(q(3))-cos(q(3)+q(4));
q3 = q(1)+q(2);
q4 = -q(2);
q_new = [q3 q4]';

== matlab function dribbel_v2/Dynamics/Subsystem1/Dynamics/Energy Loss/Energy before impact ==
  data: q input; K output; qd input
function K = Energy(q,qd)
m = 1; %kg
mH = 5; %kg
A = [cos(sum(q))-cos(q(1)) cos(sum(q));
     sin(sum(q))-sin(q(1)) sin(sum(q))];
M = zeros(2,2);
M(1,1) = mH + (3/2)*m-m*cos(q(2));
M(1,2) = (1/4)*m*(1-2*cos(q(2)));
M(2,1) = (1/4)*m*(1-2*cos(q(2)));
M(2,2) = (1/4)*m;
M = inv(M);
D = A*inv(A'*M*A)*A';
K = 0.5*(qd'*D*qd);

== matlab function dribbel_v2/Dynamics/Subsystem1/Dynamics/Energy Loss/Energy After impact ==
  data: q input; K output; qd input
function K = Energy(q,qd)
m = 1; %kg
mH = 5; %kg
A = [cos(sum(q))-cos(q(1)) cos(sum(q));
     sin(sum(q))-sin(q(1)) sin(sum(q))];
M = zeros(2,2);
M(1,1) = mH + (3/2)*m-m*cos(q(2));
M(1,2) = (1/4)*m*(1-2*cos(q(2)));
M(2,1) = (1/4)*m*(1-2*cos(q(2)));
M(2,2) = (1/4)*m;
M = inv(M);
D = A*inv(A'*M*A)*A';
K = 0.5*(qd'*D*qd);

== matlab function dribbel_v2/MATLAB Function ==
  data: q input; y output; qd input
function y = check_double_support(q,qd)
q3 = q(1); q4 = q(2); q3d = qd(1); q4d = qd(2);
y = (2*(sin(5*q3)-sin(q3))*q3d-(1/6)*sin(3*q3)*(2*q3d+q4d));

== matlab function dribbel_v2/contact_release_detection/ContactRelaease/MATLAB Function ==
  data: q input; Xdd output; qd input; qdd input
function Xdd = unconstrained_acceleration(q,qd,qdd)

A = [-cos(sum(q))+cos(q(1)) -cos(sum(q));
     -sin(sum(q))+sin(q(1)) sin(sum(q))];
A_dot = [sum(qd)*sin(sum(q))-qd(1)*sin(q(1)) sin(sum(q))*sum(qd);
         -sum(qd)*cos(sum(q))+qd(1)*cos(q(1)) -cos(sum(q))*sum(qd)];
Xdd = A*qdd+ A_dot*qd;
end

== matlab function dribbel_v2/Dynamics/torque generator/MATLAB Function1 ==
  data: q input; tau output; qd input; qdd input; m input; mH input; gamma input; g input
function tau = inverseDribbelDynamics(q,qd,qdd,m,mH,gamma, g)

M = zeros(2,2);
M(1,1) = mH + (3/2)*m-m*cos(q(2));
M(1,2) = (1/4)*m*(1-2*cos(q(2)));
M(2,1) = (1/4)*m*(1-2*cos(q(2)));
M(2,2) = (1/4)*m;

c11 = 0.0;
% c12 = 0.5*qd(1)*(-0.5*m*sin(q(2))-m*sin(q(2))-0) + 0.5*qd(2)*(-0.5*m*sin(q(2))-0.5*m*sin(q(2))-0);
% c21 = 0.5*qd(1)*(0 + 0 + m*sin(q(2))) + 0.5*qd(2)*(0 + 0 +0.5*m*sin(q(2)));
c12 = ((3/4)*qd(1)+qd(2)/2)*m*sin(q(2));
c21 = -(qd(1)/2 + qd(2)/4)*m*sin(q(2));
c22 = 0.0;

C = [c11 c12; c21 c22];

dvdq = zeros(2,1);
% dvdq(1) = -m*g*0.5*sin(q(1)-gamma) - mH*g*sin(q(1)-gamma) - m*g*sin(q(1)-gamma) + 0.5*m*g*sin(q(1)+q(2)-gamma);
dvdq(1) = -((3/2)*m*g+mH*g)*sin(q(1)-gamma)+(1/2)*m*g*sin(q(1)+q(2)-gamma);
dvdq(2) = m*g*0.5*sin(q(1)+q(2)-gamma);

tau = M*qdd+C*qd+dvdq;

== matlab function dribbel_v2/Dynamics/Subsystem1/Dynamics/forward_kinematics ==
  data: q input; c2 output
function c2 = fcn(q)
c2 = zeros(3,1);
% c2(1) = 0;
% c2(2) = q(1);
% c2(3) = q(2);

c2(1) = 0;
c2(2) = q(1)-sin(q(3))+sin(q(3)+q(4));
c2(3) = q(2)+cos(q(3))-cos(q(3)+q(4));

== matlab function dribbel_v2/Dynamics/Subsystem1/Dynamics/gravity_force/Graitational_Force ==
  data: q input size=[2,1]; dvdq output size=[2,1]; m input; mH input; gamma input; g input
function dvdq = create_grav(q,m,mH,gamma,g)

dvdq = zeros(2,1);
dvdq(1) = -((3/2)*m*g+mH*g)*sin(q(1)-gamma)+(1/2)*m*g*sin(q(1)+q(2)-gamma);
dvdq(2) = m*g*0.5*sin(q(1)+q(2)-gamma);
end

== matlab function dribbel_v2/Dynamics/Subsystem/Dynamics1/C_matrix/C_matrix ==
  data: q input size=[2,1]; C output size=[2,2]; qd input size=[2,1]; m input
function C = create_C(q, qd,m)

c11 = 0.0;
c12 = ((3/4)*qd(1)+qd(2)/2)*m*sin(q(2));
c21 = -(qd(1)/2 + qd(2)/4)*m*sin(q(2));
c22 = 0.0;
C = [c11 c12; c21 c22];

end

== matlab function dribbel_v2/Dynamics/Subsystem/Dynamics1/forward_kinematics ==
  data: q input; c2 output
function c2 = fcn(q)
c2 = zeros(3,1);
% c2(1) = 0;
% c2(2) = q(1);
% c2(3) = q(2);

c2(1) = 0;
c2(2) = q(1)-sin(q(3))+sin(q(3)+q(4));
c2(3) = q(2)+cos(q(3))-cos(q(3)+q(4));

== matlab function dribbel_v2/Dynamics/Subsystem1/Dynamics/mass_matrix/Mass_Matrix ==
  data: q input size=[2,1]; M output size=[2,2]; M_inv output; m input; mH input
function [M,M_inv] = create_mass(q,m,mH)
% mH = 0.1;
% m = 0.05;

M = zeros(2,2);
M(1,1) = mH + (3/2)*m-m*cos(q(2));
M(1,2) = (1/4)*m*(1-2*cos(q(2)));
M(2,1) = (1/4)*m*(1-2*cos(q(2)));
M(2,2) = (1/4)*m;
M_inv = inv(M);
end

== matlab function dribbel_v2/Dynamics/Subsystem/Dynamics1/gravity_force/Graitational_Force ==
  data: q input size=[2,1]; dvdq output size=[2,1]; m input; mH input; gamma input; g input
function dvdq = create_grav(q,m,mH,gamma,g)

dvdq = zeros(2,1);
dvdq(1) = -((3/2)*m*g+mH*g)*sin(q(1)-gamma)+(1/2)*m*g*sin(q(1)+q(2)-gamma);
dvdq(2) = m*g*0.5*sin(q(1)+q(2)-gamma);
end

== matlab function dribbel_v2/Dynamics/Subsystem/Dynamics1/mass_matrix/Mass_Matrix ==
  data: q input size=[2,1]; M output size=[2,2]; M_inv output; m input; mH input
function [M,M_inv] = create_mass(q,m,mH)
% mH = 0.1;
% m = 0.05;

M = zeros(2,2);
M(1,1) = mH + (3/2)*m-m*cos(q(2));
M(1,2) = (1/4)*m*(1-2*cos(q(2)));
M(2,1) = (1/4)*m*(1-2*cos(q(2)));
M(2,2) = (1/4)*m;
M_inv = inv(M);
end
